simulink model "passThrough"  (R2020a)
settings: Solver=FixedStepDiscrete  StartTime=0.0  StopTime=100  RelTol=1e-3
InitFcn:
  | xlEvaluateHDLBlocks('passThrough')
undefined symbols (not defined in the file): S, xc7vx485tffg1157
libraries: ModelComposer x4, xbsIndex_r4 x2, simulink x1, dspsrcs4 x1
settings Model: Creator=shirazi  LastModifiedBy=abehbood
settings SFSimCC: CustomCodeUndefinedFunction=UseInterfaceOnly

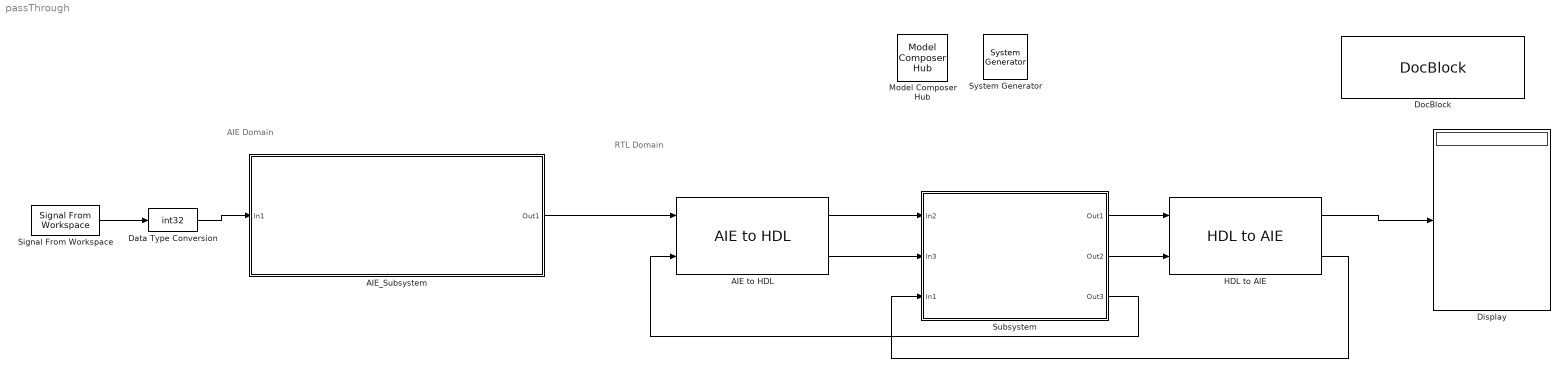
== system passThrough ==
  note: AIE Domain
  note: RTL Domain
  " System Generator" : xbsIndex_r4/ System Generator  Tag=genX  xilinxfamily=versalaicore  part=xcvc1902  speed=-2MP-e-S  package=vsva2197  synthesis_tool=Vivado  clock_wrapper=Clock Enables  directory=./netlist  proj_type=Vivado  Synth_file=Vivado Synthesis Defaults  Impl_file=Vivado Implementation Defaults  testbench=off  simulink_period=1  sysclk_period=10  dcm_input_clock_period=10  incr_netlist=off  trim_vbits=Everywhere in SubSystem  dbl_ovrd=According to Block Masks  core_generation=According to Block Masks  run_coregen=off  deprecated_control=off  eval_field=0  block_type=sysgen
  AIE to HDL : ModelComposer/AIE to HDL  OutDataType=int32  OutSampleTime=1
  AIE_Subsystem : Subsystem
  Data Type Conversion : DataTypeConversion  OutDataTypeStr=int32
  Display : Display
  DocBlock : simulink/Model-Wide Utilities/DocBlock  DocumentType=Text  mask(DocBlock){}
      content=|
      | ///////////////////////////////////////////////////////////////////////////
      | // Copyright 2021 Xilinx
      | //
      | // Licensed under the Apache License, Version 2.0 (the "License");
      | // you may not use this file except in compliance with the License.
      | // You may obtain a copy of the License at
      | //
      | // http://www.apache.org/licenses/LICENSE-2.0
      | //
      | // Unless required by applicable law or agreed to in writing, software
      | // distributed under the License is distributed on an "AS IS" BASIS,
      | // WITHOUT WARRANTIES OR CONDITIONS OF ANY KIND, either express or implied.
      | // See the License for the specific language governing permissions and
      | // limitations under the License.
      | ///////////////////////////////////////////////////////////////////////////
      mask Display:
      | xmcDrawBlockIcon();
      | disp(['{\fontsize{10pt}(c) Copyright 2021' ' Xilinx, Inc.}\newline \newline '],'texmode','on');
      | disp('{\fontsize{10pt}Licensed under the Apache License 2.0}','texmode','on');
      | disp('\newline \newline \newline{\fontsize{10pt}Double Click for Copyright Notice}','texmode','on');
  HDL to AIE : ModelComposer/HDL to AIE  OutDataType=int32  OutSampleTime=1  SamplesPerFrame=8  TreadySampleTime=1
  Model Composer Hub : ModelComposer/Model Composer Hub  CodeGeneration=off  SubsystemName=AIE_Subsystem  TargetDirectory=./aie_code  ExportType=AI Engines  IpVendor=xilinx.com  IpLibrary=hls  IpVersion=1.0  IpHWLanguage=Verilog  AieCompilerOptions={}  CreateTestbench=on  TestbenchStackSize=10  RunAieSim=on  AieSimTimeout=50000  RunAieSimProfiling=off  LaunchVitisAnalyzer=off  PlotOutput=off  RunX86Sim=on  X86SimTimeout=10  GenHwImage=off  PlatformType=Not Specified  ProjDevice=xc7vx485tffg1157-1  ProjDevicePart=xc7vx485tffg1157-1  SamplePeriod=-1  ClockFrequency=200  DataPathParallelism=1
  Signal From Workspace : dspsrcs4/Signal From Workspace  X=1:100  Ts=1  nsamps=8  OutputAfterFinalValue=Cyclic repetition  ignoreOrWarnInputAndFrameLengths=off  OutputFrames=off
  Subsystem : Subsystem
  wires:
  Signal From Workspace/1 -> Data Type Conversion/1
  HDL to AIE/1 -> Display/1
  Subsystem/1(Out1) -> HDL to AIE/1
  AIE to HDL/1 -> Subsystem/1(In2)
  Subsystem/2(Out2) -> HDL to AIE/2
  AIE to HDL/2 -> Subsystem/2(In3)
  HDL to AIE/2 -> Subsystem/3(In1)
  Subsystem/3(Out3) -> AIE to HDL/2
  Data Type Conversion/1 -> AIE_Subsystem/1(In1)
  AIE_Subsystem/1(Out1) -> AIE to HDL/1

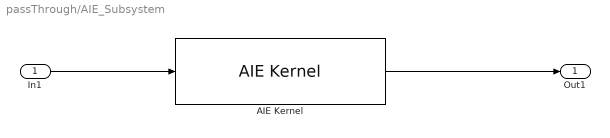
== system passThrough/AIE_Subsystem ==
  In1 : Inport
  AIE Kernel : ModelComposer/AIE Kernel  KernelAllAttrs=s[12;12;9;9;19;14;21;23;24;21;12;24;26;26;26;27;28;9;21;23;23;23;24;25;14;19;19;29]@FunctionNameDeclFileNamePortNamesPortTypesPortSerializedTypesPortDirectionsPortWindowSizeEnablesPortWindowMarginEnablesPortSynchronicityEnablesPortSignalSizeEnablesFunctionDeclFunctionTemplateSpecKindFunctionTemplateParamNamesFunctionTemplateParamKindsFunctionTemplateParamTypesFunctionTemplateParamValuesFunctionTemplateParamEnablesClassDeclClassTemplateSpecKindClassTemplateParamNamesClassTemplateParamKindsClassTemplateParamTypesClassTemplateParamValuesClassTemplateParamEnablesClassCtorDeclsClassCtorParamNamesClassCtorParamTypesClassCtorParamSerializedTypes[1 1]@C[28 1]@t8@mysquaret16@../../mysquare.hC[2 1]@t3@in1t4@out1C[2 1]@t20@input_window_int32 *t21@output_window_int32 *C[2 1]@t30@{P{Tinput_window{1{t{Bi32}}}}}t31@{P{Toutput_window{1{t{Bi32}}}}}C[2 1]@t5@inputt6@outputC[2 1]@l1@l1@C[2 1]@l1@l0@C[2 1]@l1@l1@C[2 1]@l0@l0@t67@void mysquare(input_window_int32 * in1, output_window_int32 * out1)t4@nonee[0 1]@e[0 1]@e[0 1]@e[0 1]@e[0 1]@nne[0 1]@e[0 1]@e[0 1]@e[0 1]@e[0 1]@e[0 1]@e[0 1]@e[0 1]@e[0 1]@  PortNames={'in1'; 'out1'}  PortSerializedTypes={'{P{Tinput_window{1{t{Bi32}}}}}'; '{P{Toutput_window{1{t{Bi32}}}}}'}  PortWindowSizes={8.000000000000000000e+00; 8.000000000000000000e+00}  PortWindowMargins={0.000000000000000000e+00; 0.000000000000000000e+00}  PortSynchronicities={'sync'; 'sync'}  PortSignalSizes={0.000000000000000000e+00; 0.000000000000000000e+00}  FunctionTemplateSpecKind=none  FunctionTemplateParamNames={}  FunctionTemplateParamKinds={}  FunctionTemplateParamTypes={}  FunctionTemplateParamValues={}  FunctionIndex=1  FunctionTabVisible=on  FunctionTemplateParamsVisible=off  FunctionDeclTypeOptions=C[1 1]@t70@void mysquare(input_window_int32 * _arg0, output_window_int32 * _arg1)  FunctionDecl=void mysquare(input_window_int32 * _arg0, output_window_int32 * _arg1)  FunctionTemplateParams={}  FunctionTemplateParamsEnables={}  PortAttrs={ 'Input', '_arg0', 'input_window_int32 *', '8', '0', 'sync', ''; 'Output', '_arg1', 'output_window_int32 *', '8', '', 'sync', '' }  PortAttrsEnables={'off', 'off', 'off', 'on', 'on', 'on', 'off';'off', 'off', 'off', 'on', 'off', 'on', 'off'}  KernelHeaderFile=mysquare.h  KernelFunction=mysquare  KernelSourceFile=mysquare.cc  KernelSearchPaths={}  PreProcOptions={}  CoreRuntimeRatio=0.9  KernelLocSpec=off  ColRowLocation=[0 0]  blockJsonConstraints="{\"type\":\"constraint\",\"constraintType\":\"coreUtilization\",\"sid\":\"282\",\"lhs\":{\"type\":\"runtimeRatio\",\"args\":{\"type\":\"kernel\",\"name\":\"ModelComposer/AIE Kernel\",\"sid\":\"282\"}},\"rhs\":{\"type\":\"evaluable\",\"expr\":\"0.9\",\"value\":0.9},\"equality\":true}"  deprecateConstraints=0
  Out1 : Outport
  wires:
  In1/1 -> AIE Kernel/1
  AIE Kernel/1 -> Out1/1

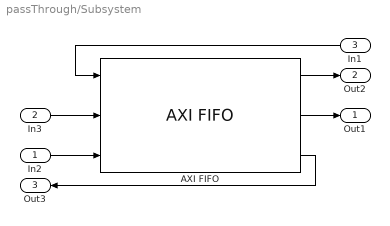
== system passThrough/Subsystem ==
  In2 : Inport
  In3 : Inport  Port=2
  In1 : Inport  Port=3
  AXI FIFO : xbsIndex_r4/AXI FIFO  input_depth_axis=1K  actual_fifo_depth_label=1026  enable_tdata=on  enable_tdest=off  enable_tstrb=off  enable_tready=on  enable_tid=off  enable_tuser=off  enable_tkeep=off  enable_tlast=off  has_aresetn=off  enable_data_counts_axis=off  fifo_implementation_type_axis=Common Clock Block RAM  trim_axipin_name=off  programmable_full_type_axis=Full  full_threshold_assert_value_axis=0  programmable_empty_type_axis=Empty  empty_threshold_assert_value_axis=1022  underflow_flag_axi=0  underflow_sense_axi=Active High  overflow_flag_axi=0  overflow_sense_axi=Active High  simulation_type=fast_sim  block_type=axi_fifo
  Out1 : Outport
  Out2 : Outport  Port=2
  Out3 : Outport  Port=3
  wires:
  AXI FIFO/2 -> Out1/1
  AXI FIFO/1 -> Out2/1
  In1/1 -> AXI FIFO/1
  AXI FIFO/3 -> Out3/1
  In2/1 -> AXI FIFO/3
  In3/1 -> AXI FIFO/2
